simulink model "model3"  (R2018b)
settings: Solver=VariableStepAuto  StartTime=0.0  StopTime=15  RelTol=1e-3
settings Model: Creator=HYJ  LastModifiedBy=HYJ

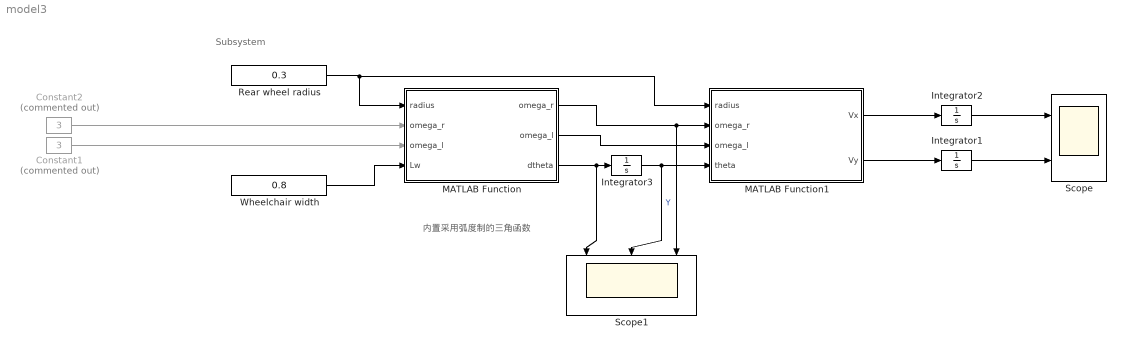
== system model3 ==
  note: Subsystem
  note: 内置采用弧度制的三角函数
  Constant1 : Constant  Commented=on  Value=3
  Constant2 : Constant  Commented=on  Value=3
  Integrator1 : Integrator
  Integrator2 : Integrator
  Integrator3 : Integrator
  MATLAB Function : MATLAB Function  TreatAsAtomicUnit=on
  MATLAB Function1 : MATLAB Function  TreatAsAtomicUnit=on
  Rear wheel radius : Constant  Value=0.3
  Scope : Scope  NumInputPorts=2
  Scope1 : Scope  NumInputPorts=3
  Wheelchair width : Constant  Value=0.8
  wires:
  Integrator2/1 -> Scope/1
  Integrator1/1 -> Scope/2
  Constant2/1 -> MATLAB Function/2("omega_r ")
  Constant1/1 -> MATLAB Function/3("omega_l ")
  Wheelchair width/1 -> MATLAB Function/4(Lw)
  Rear wheel radius/1 -> MATLAB Function1/1(radius), MATLAB Function/1(radius)
  MATLAB Function/1(omega_r) -> MATLAB Function1/2(omega_r), Scope1/3
  Integrator3/1 -> Scope1/2, MATLAB Function1/4(theta)  "Y"
  MATLAB Function/2(omega_l) -> MATLAB Function1/3(omega_l)
  MATLAB Function1/2(Vy) -> Integrator1/1
  MATLAB Function/3(dtheta) -> Scope1/1, Integrator3/1
  MATLAB Function1/1(Vx) -> Integrator2/1

== matlab function model3/MATLAB Function1 ==
  data: radius input; omega_r input; omega_l input; theta input; Vx output; Vy output
function [Vx, Vy]  = MPW_velocity(radius, omega_r, omega_l, theta)

Vx = 0.5 * radius * cos(theta) * (omega_r + omega_l);
Vy = 0.5 * radius * sin(theta) * (omega_r + omega_l);

end

== matlab function model3/MATLAB Function ==
  data: omega_r output; omega_l output; radius input; omega_r input; omega_l input; Lw input; dtheta output
function [omega_r,omega_l,dtheta]  = MPW_main(radius, omega_r, omega_l, Lw)

dtheta = 2 * radius * ((omega_r/Lw) - (omega_l/Lw));
omega_r = omega_r;
omega_l = omega_l;
end
